simulink model "IOControls"  (R2019b)
settings: configuration reference "ConfigSet_IOControls_Reference" (kept outside this file)
model workspace (MAT data in the model file):
  SampleTime = 0.05
libraries: IOStateMachinesLib x274, SignalGeneratorsLib x1, simulink x1
(part 5 of 10)

== system IOControls/ForEachVehicle/IOControls/Non-CabControl/CircuitBreakersofEDB/BCGCB ==
  note: States:
      | Tripped
      | Set
  MCBControl : Inport  OutDataTypeStr=Bus: BD_IOControls_In_MCBControl
  Initialise : Inport  Port=2
  BCGCB-MCB : IOStateMachinesLib/MCB  InitSource=internal  InitState=InitState  OffStateValue=OffStateValue  OnStateValue=OnStateValue
      settings: SourceProductName=IO State Machines
  Bus Selector : BusSelector  OutputSignals=Value,Mode,InitVal,InternalRequest,Inhibit,TripRequest
  InputState : Outport  VectorParamsAs1DForOutWhenUnconnected=off
  MCBTripState : Outport  Port=2  VectorParamsAs1DForOutWhenUnconnected=off
  wires:
  BCGCB-MCB/2 -> MCBTripState/1
  Bus Selector/6 -> BCGCB-MCB/7  "<TripRequest>"
  MCBControl/1 -> Bus Selector/1
  Bus Selector/1 -> BCGCB-MCB/1  "<Value>"
  Bus Selector/2 -> BCGCB-MCB/2  "<Mode>"
  Bus Selector/3 -> BCGCB-MCB/3  "<InitVal>"
  Bus Selector/4 -> BCGCB-MCB/5  "<InternalRequest>"
  Bus Selector/5 -> BCGCB-MCB/6  "<Inhibit>"
  BCGCB-MCB/1 -> InputState/1
  Initialise/1 -> BCGCB-MCB/4

== system IOControls/ForEachVehicle/IOControls/Non-CabControl/CircuitBreakersofEDB/BECUCB1 ==
  note: States:
      | Tripped
      | Set
  MCBControl : Inport  OutDataTypeStr=Bus: BD_IOControls_In_MCBControl
  Initialise : Inport  Port=2
  BECUCB1-MCB : IOStateMachinesLib/MCB  InitSource=internal  InitState=InitState  OffStateValue=OffStateValue  OnStateValue=OnStateValue
      settings: SourceProductName=IO State Machines
  Bus Selector : BusSelector  OutputSignals=Value,Mode,InitVal,InternalRequest,Inhibit,TripRequest
  InputState : Outport  VectorParamsAs1DForOutWhenUnconnected=off
  MCBTripState : Outport  Port=2  VectorParamsAs1DForOutWhenUnconnected=off
  wires:
  BECUCB1-MCB/2 -> MCBTripState/1
  Bus Selector/6 -> BECUCB1-MCB/7  "<TripRequest>"
  MCBControl/1 -> Bus Selector/1
  Bus Selector/1 -> BECUCB1-MCB/1  "<Value>"
  Bus Selector/2 -> BECUCB1-MCB/2  "<Mode>"
  Bus Selector/3 -> BECUCB1-MCB/3  "<InitVal>"
  Bus Selector/4 -> BECUCB1-MCB/5  "<InternalRequest>"
  Bus Selector/5 -> BECUCB1-MCB/6  "<Inhibit>"
  BECUCB1-MCB/1 -> InputState/1
  Initialise/1 -> BECUCB1-MCB/4

== system IOControls/ForEachVehicle/IOControls/Non-CabControl/CircuitBreakersofEDB/BECUCB2 ==
  note: States:
      | Tripped
      | Set
  MCBControl : Inport  OutDataTypeStr=Bus: BD_IOControls_In_MCBControl
  Initialise : Inport  Port=2
  BECUCB2-MCB : IOStateMachinesLib/MCB  InitSource=internal  InitState=InitState  OffStateValue=OffStateValue  OnStateValue=OnStateValue
      settings: SourceProductName=IO State Machines
  Bus Selector : BusSelector  OutputSignals=Value,Mode,InitVal,InternalRequest,Inhibit,TripRequest
  InputState : Outport  VectorParamsAs1DForOutWhenUnconnected=off
  MCBTripState : Outport  Port=2  VectorParamsAs1DForOutWhenUnconnected=off
  wires:
  BECUCB2-MCB/2 -> MCBTripState/1
  Bus Selector/6 -> BECUCB2-MCB/7  "<TripRequest>"
  MCBControl/1 -> Bus Selector/1
  Bus Selector/1 -> BECUCB2-MCB/1  "<Value>"
  Bus Selector/2 -> BECUCB2-MCB/2  "<Mode>"
  Bus Selector/3 -> BECUCB2-MCB/3  "<InitVal>"
  Bus Selector/4 -> BECUCB2-MCB/5  "<InternalRequest>"
  Bus Selector/5 -> BECUCB2-MCB/6  "<Inhibit>"
  BECUCB2-MCB/1 -> InputState/1
  Initialise/1 -> BECUCB2-MCB/4

== system IOControls/ForEachVehicle/IOControls/Non-CabControl/CircuitBreakersofEDB/BECUCB3 ==
  note: States:
      | Tripped
      | Set
  MCBControl : Inport  OutDataTypeStr=Bus: BD_IOControls_In_MCBControl
  Initialise : Inport  Port=2
  BECUCB3-MCB : IOStateMachinesLib/MCB  InitSource=internal  InitState=InitState  OffStateValue=OffStateValue  OnStateValue=OnStateValue
      settings: SourceProductName=IO State Machines
  Bus Selector : BusSelector  OutputSignals=Value,Mode,InitVal,InternalRequest,Inhibit,TripRequest
  InputState : Outport  VectorParamsAs1DForOutWhenUnconnected=off
  MCBTripState : Outport  Port=2  VectorParamsAs1DForOutWhenUnconnected=off
  wires:
  BECUCB3-MCB/2 -> MCBTripState/1
  Bus Selector/6 -> BECUCB3-MCB/7  "<TripRequest>"
  MCBControl/1 -> Bus Selector/1
  Bus Selector/1 -> BECUCB3-MCB/1  "<Value>"
  Bus Selector/2 -> BECUCB3-MCB/2  "<Mode>"
  Bus Selector/3 -> BECUCB3-MCB/3  "<InitVal>"
  Bus Selector/4 -> BECUCB3-MCB/5  "<InternalRequest>"
  Bus Selector/5 -> BECUCB3-MCB/6  "<Inhibit>"
  BECUCB3-MCB/1 -> InputState/1
  Initialise/1 -> BECUCB3-MCB/4

== system IOControls/ForEachVehicle/IOControls/Non-CabControl/CircuitBreakersofEDB/BLCB ==
  note: States:
      | Tripped
      | Set
  MCBControl : Inport  OutDataTypeStr=Bus: BD_IOControls_In_MCBControl
  Initialise : Inport  Port=2
  BLCB-MCB : IOStateMachinesLib/MCB  InitSource=internal  InitState=InitState  OffStateValue=OffStateValue  OnStateValue=OnStateValue
      settings: SourceProductName=IO State Machines
  Bus Selector : BusSelector  OutputSignals=Value,Mode,InitVal,InternalRequest,Inhibit,TripRequest
  InputState : Outport  VectorParamsAs1DForOutWhenUnconnected=off
  MCBTripState : Outport  Port=2  VectorParamsAs1DForOutWhenUnconnected=off
  wires:
  BLCB-MCB/2 -> MCBTripState/1
  Bus Selector/6 -> BLCB-MCB/7  "<TripRequest>"
  MCBControl/1 -> Bus Selector/1
  Bus Selector/1 -> BLCB-MCB/1  "<Value>"
  Bus Selector/2 -> BLCB-MCB/2  "<Mode>"
  Bus Selector/3 -> BLCB-MCB/3  "<InitVal>"
  Bus Selector/4 -> BLCB-MCB/5  "<InternalRequest>"
  Bus Selector/5 -> BLCB-MCB/6  "<Inhibit>"
  BLCB-MCB/1 -> InputState/1
  Initialise/1 -> BLCB-MCB/4

== system IOControls/ForEachVehicle/IOControls/Non-CabControl/CircuitBreakersofEDB/C1CB ==
  note: States:
      | Tripped
      | Set
  MCBControl : Inport  OutDataTypeStr=Bus: BD_IOControls_In_MCBControl
  Initialise : Inport  Port=2
  Bus Selector : BusSelector  OutputSignals=Value,Mode,InitVal,InternalRequest,Inhibit,TripRequest
  C1CB-MCB : IOStateMachinesLib/MCB  InitSource=internal  InitState=InitState  OffStateValue=OffStateValue  OnStateValue=OnStateValue
      settings: SourceProductName=IO State Machines
  InputState : Outport  VectorParamsAs1DForOutWhenUnconnected=off
  MCBTripState : Outport  Port=2  VectorParamsAs1DForOutWhenUnconnected=off
  wires:
  C1CB-MCB/2 -> MCBTripState/1
  Bus Selector/6 -> C1CB-MCB/7  "<TripRequest>"
  MCBControl/1 -> Bus Selector/1
  Bus Selector/1 -> C1CB-MCB/1  "<Value>"
  Bus Selector/2 -> C1CB-MCB/2  "<Mode>"
  Bus Selector/3 -> C1CB-MCB/3  "<InitVal>"
  Bus Selector/4 -> C1CB-MCB/5  "<InternalRequest>"
  Bus Selector/5 -> C1CB-MCB/6  "<Inhibit>"
  C1CB-MCB/1 -> InputState/1
  Initialise/1 -> C1CB-MCB/4

== system IOControls/ForEachVehicle/IOControls/Non-CabControl/CircuitBreakersofEDB/CBFCB ==
  note: States:
      | Tripped
      | Set
  MCBControl : Inport  OutDataTypeStr=Bus: BD_IOControls_In_MCBControl
  Initialise : Inport  Port=2
  Bus Selector : BusSelector  OutputSignals=Value,Mode,InitVal,InternalRequest,Inhibit,TripRequest
  CBFCB-MCB : IOStateMachinesLib/MCB  InitSource=internal  InitState=InitState  OffStateValue=OffStateValue  OnStateValue=OnStateValue
      settings: SourceProductName=IO State Machines
  InputState : Outport  VectorParamsAs1DForOutWhenUnconnected=off
  MCBTripState : Outport  Port=2  VectorParamsAs1DForOutWhenUnconnected=off
  wires:
  CBFCB-MCB/2 -> MCBTripState/1
  Bus Selector/6 -> CBFCB-MCB/7  "<TripRequest>"
  MCBControl/1 -> Bus Selector/1
  Bus Selector/1 -> CBFCB-MCB/1  "<Value>"
  Bus Selector/2 -> CBFCB-MCB/2  "<Mode>"
  Bus Selector/3 -> CBFCB-MCB/3  "<InitVal>"
  Bus Selector/4 -> CBFCB-MCB/5  "<InternalRequest>"
  Bus Selector/5 -> CBFCB-MCB/6  "<Inhibit>"
  CBFCB-MCB/1 -> InputState/1
  Initialise/1 -> CBFCB-MCB/4

== system IOControls/ForEachVehicle/IOControls/Non-CabControl/CircuitBreakersofEDB/CBFCCB ==
  note: States:
      | Tripped
      | Set
  MCBControl : Inport  OutDataTypeStr=Bus: BD_IOControls_In_MCBControl
  Initialise : Inport  Port=2
  Bus Selector : BusSelector  OutputSignals=Value,Mode,InitVal,InternalRequest,Inhibit,TripRequest
  CBFCCB-MCB : IOStateMachinesLib/MCB  InitSource=internal  InitState=InitState  OffStateValue=OffStateValue  OnStateValue=OnStateValue
      settings: SourceProductName=IO State Machines
  InputState : Outport  VectorParamsAs1DForOutWhenUnconnected=off
  MCBTripState : Outport  Port=2  VectorParamsAs1DForOutWhenUnconnected=off
  wires:
  CBFCCB-MCB/2 -> MCBTripState/1
  Bus Selector/6 -> CBFCCB-MCB/7  "<TripRequest>"
  MCBControl/1 -> Bus Selector/1
  Bus Selector/1 -> CBFCCB-MCB/1  "<Value>"
  Bus Selector/2 -> CBFCCB-MCB/2  "<Mode>"
  Bus Selector/3 -> CBFCCB-MCB/3  "<InitVal>"
  Bus Selector/4 -> CBFCCB-MCB/5  "<InternalRequest>"
  Bus Selector/5 -> CBFCCB-MCB/6  "<Inhibit>"
  CBFCCB-MCB/1 -> InputState/1
  Initialise/1 -> CBFCCB-MCB/4

== system IOControls/ForEachVehicle/IOControls/Non-CabControl/CircuitBreakersofEDB/CBTCCB1 ==
  note: States:
      | Tripped
      | Set
  MCBControl : Inport  OutDataTypeStr=Bus: BD_IOControls_In_MCBControl
  Initialise : Inport  Port=2
  Bus Selector : BusSelector  OutputSignals=Value,Mode,InitVal,InternalRequest,Inhibit,TripRequest
  CBTCCB1-MCB : IOStateMachinesLib/MCB  InitSource=internal  InitState=InitState  OffStateValue=OffStateValue  OnStateValue=OnStateValue
      settings: SourceProductName=IO State Machines
  InputState : Outport  VectorParamsAs1DForOutWhenUnconnected=off
  MCBTripState : Outport  Port=2  VectorParamsAs1DForOutWhenUnconnected=off
  wires:
  CBTCCB1-MCB/2 -> MCBTripState/1
  Bus Selector/6 -> CBTCCB1-MCB/7  "<TripRequest>"
  MCBControl/1 -> Bus Selector/1
  Bus Selector/1 -> CBTCCB1-MCB/1  "<Value>"
  Bus Selector/2 -> CBTCCB1-MCB/2  "<Mode>"
  Bus Selector/3 -> CBTCCB1-MCB/3  "<InitVal>"
  Bus Selector/4 -> CBTCCB1-MCB/5  "<InternalRequest>"
  Bus Selector/5 -> CBTCCB1-MCB/6  "<Inhibit>"
  CBTCCB1-MCB/1 -> InputState/1
  Initialise/1 -> CBTCCB1-MCB/4

== system IOControls/ForEachVehicle/IOControls/Non-CabControl/CircuitBreakersofEDB/CCNVIO1CB ==
  note: States:
      | Tripped
      | Set
  MCBControl : Inport  OutDataTypeStr=Bus: BD_IOControls_In_MCBControl
  Initialise : Inport  Port=2
  Bus Selector : BusSelector  OutputSignals=Value,Mode,InitVal,InternalRequest,Inhibit,TripRequest
  CCNVIO1CB-MCB : IOStateMachinesLib/MCB  InitSource=internal  InitState=InitState  OffStateValue=OffStateValue  OnStateValue=OnStateValue
      settings: SourceProductName=IO State Machines
  InputState : Outport  VectorParamsAs1DForOutWhenUnconnected=off
  MCBTripState : Outport  Port=2  VectorParamsAs1DForOutWhenUnconnected=off
  wires:
  CCNVIO1CB-MCB/2 -> MCBTripState/1
  Bus Selector/6 -> CCNVIO1CB-MCB/7  "<TripRequest>"
  MCBControl/1 -> Bus Selector/1
  Bus Selector/1 -> CCNVIO1CB-MCB/1  "<Value>"
  Bus Selector/2 -> CCNVIO1CB-MCB/2  "<Mode>"
  Bus Selector/3 -> CCNVIO1CB-MCB/3  "<InitVal>"
  Bus Selector/4 -> CCNVIO1CB-MCB/5  "<InternalRequest>"
  Bus Selector/5 -> CCNVIO1CB-MCB/6  "<Inhibit>"
  CCNVIO1CB-MCB/1 -> InputState/1
  Initialise/1 -> CCNVIO1CB-MCB/4

== system IOControls/ForEachVehicle/IOControls/Non-CabControl/CircuitBreakersofEDB/CDUCB ==
  note: States:
      | Tripped
      | Set
  MCBControl : Inport  OutDataTypeStr=Bus: BD_IOControls_In_MCBControl
  Initialise : Inport  Port=2
  Bus Selector : BusSelector  OutputSignals=Value,Mode,InitVal,InternalRequest,Inhibit,TripRequest
  CDUCB-MCB : IOStateMachinesLib/MCB  InitSource=internal  InitState=InitState  OffStateValue=OffStateValue  OnStateValue=OnStateValue
      settings: SourceProductName=IO State Machines
  InputState : Outport  VectorParamsAs1DForOutWhenUnconnected=off
  MCBTripState : Outport  Port=2  VectorParamsAs1DForOutWhenUnconnected=off
  wires:
  CDUCB-MCB/2 -> MCBTripState/1
  Bus Selector/6 -> CDUCB-MCB/7  "<TripRequest>"
  MCBControl/1 -> Bus Selector/1
  Bus Selector/1 -> CDUCB-MCB/1  "<Value>"
  Bus Selector/2 -> CDUCB-MCB/2  "<Mode>"
  Bus Selector/3 -> CDUCB-MCB/3  "<InitVal>"
  Bus Selector/4 -> CDUCB-MCB/5  "<InternalRequest>"
  Bus Selector/5 -> CDUCB-MCB/6  "<Inhibit>"
  CDUCB-MCB/1 -> InputState/1
  Initialise/1 -> CDUCB-MCB/4

== system IOControls/ForEachVehicle/IOControls/Non-CabControl/CircuitBreakersofEDB/CECB ==
  note: States:
      | Tripped
      | Set
  MCBControl : Inport  OutDataTypeStr=Bus: BD_IOControls_In_MCBControl
  Initialise : Inport  Port=2
  Bus Selector : BusSelector  OutputSignals=Value,Mode,InitVal,InternalRequest,Inhibit,TripRequest
  CECB-MCB : IOStateMachinesLib/MCB  InitSource=internal  InitState=InitState  OffStateValue=OffStateValue  OnStateValue=OnStateValue
      settings: SourceProductName=IO State Machines
  InputState : Outport  VectorParamsAs1DForOutWhenUnconnected=off
  MCBTripState : Outport  Port=2  VectorParamsAs1DForOutWhenUnconnected=off
  wires:
  CECB-MCB/2 -> MCBTripState/1
  Bus Selector/6 -> CECB-MCB/7  "<TripRequest>"
  MCBControl/1 -> Bus Selector/1
  Bus Selector/1 -> CECB-MCB/1  "<Value>"
  Bus Selector/2 -> CECB-MCB/2  "<Mode>"
  Bus Selector/3 -> CECB-MCB/3  "<InitVal>"
  Bus Selector/4 -> CECB-MCB/5  "<InternalRequest>"
  Bus Selector/5 -> CECB-MCB/6  "<Inhibit>"
  CECB-MCB/1 -> InputState/1
  Initialise/1 -> CECB-MCB/4

== system IOControls/ForEachVehicle/IOControls/Non-CabControl/CircuitBreakersofEDB/CELCB ==
  note: States:
      | Tripped
      | Set
  MCBControl : Inport  OutDataTypeStr=Bus: BD_IOControls_In_MCBControl
  Initialise : Inport  Port=2
  Bus Selector : BusSelector  OutputSignals=Value,Mode,InitVal,InternalRequest,Inhibit,TripRequest
  CELCB-MCB : IOStateMachinesLib/MCB  InitSource=internal  InitState=InitState  OffStateValue=OffStateValue  OnStateValue=OnStateValue
      settings: SourceProductName=IO State Machines
  InputState : Outport  VectorParamsAs1DForOutWhenUnconnected=off
  MCBTripState : Outport  Port=2  VectorParamsAs1DForOutWhenUnconnected=off
  wires:
  CELCB-MCB/2 -> MCBTripState/1
  Bus Selector/6 -> CELCB-MCB/7  "<TripRequest>"
  MCBControl/1 -> Bus Selector/1
  Bus Selector/1 -> CELCB-MCB/1  "<Value>"
  Bus Selector/2 -> CELCB-MCB/2  "<Mode>"
  Bus Selector/3 -> CELCB-MCB/3  "<InitVal>"
  Bus Selector/4 -> CELCB-MCB/5  "<InternalRequest>"
  Bus Selector/5 -> CELCB-MCB/6  "<Inhibit>"
  CELCB-MCB/1 -> InputState/1
  Initialise/1 -> CELCB-MCB/4

== system IOControls/ForEachVehicle/IOControls/Non-CabControl/CircuitBreakersofEDB/CICB ==
  note: States:
      | Tripped
      | Set
  MCBControl : Inport  OutDataTypeStr=Bus: BD_IOControls_In_MCBControl
  Initialise : Inport  Port=2
  Bus Selector : BusSelector  OutputSignals=Value,Mode,InitVal,InternalRequest,Inhibit,TripRequest
  CICB-MCB : IOStateMachinesLib/MCB  InitSource=internal  InitState=InitState  OffStateValue=OffStateValue  OnStateValue=OnStateValue
      settings: SourceProductName=IO State Machines
  InputState : Outport  VectorParamsAs1DForOutWhenUnconnected=off
  MCBTripState : Outport  Port=2  VectorParamsAs1DForOutWhenUnconnected=off
  wires:
  CICB-MCB/2 -> MCBTripState/1
  Bus Selector/6 -> CICB-MCB/7  "<TripRequest>"
  MCBControl/1 -> Bus Selector/1
  Bus Selector/1 -> CICB-MCB/1  "<Value>"
  Bus Selector/2 -> CICB-MCB/2  "<Mode>"
  Bus Selector/3 -> CICB-MCB/3  "<InitVal>"
  Bus Selector/4 -> CICB-MCB/5  "<InternalRequest>"
  Bus Selector/5 -> CICB-MCB/6  "<Inhibit>"
  CICB-MCB/1 -> InputState/1
  Initialise/1 -> CICB-MCB/4

== system IOControls/ForEachVehicle/IOControls/Non-CabControl/CircuitBreakersofEDB/CILCB ==
  note: States:
      | Tripped
      | Set
  MCBControl : Inport  OutDataTypeStr=Bus: BD_IOControls_In_MCBControl
  Initialise : Inport  Port=2
  Bus Selector : BusSelector  OutputSignals=Value,Mode,InitVal,InternalRequest,Inhibit,TripRequest
  CILCB-MCB : IOStateMachinesLib/MCB  InitSource=internal  InitState=InitState  OffStateValue=OffStateValue  OnStateValue=OnStateValue
      settings: SourceProductName=IO State Machines
  InputState : Outport  VectorParamsAs1DForOutWhenUnconnected=off
  MCBTripState : Outport  Port=2  VectorParamsAs1DForOutWhenUnconnected=off
  wires:
  CILCB-MCB/2 -> MCBTripState/1
  Bus Selector/6 -> CILCB-MCB/7  "<TripRequest>"
  MCBControl/1 -> Bus Selector/1
  Bus Selector/1 -> CILCB-MCB/1  "<Value>"
  Bus Selector/2 -> CILCB-MCB/2  "<Mode>"
  Bus Selector/3 -> CILCB-MCB/3  "<InitVal>"
  Bus Selector/4 -> CILCB-MCB/5  "<InternalRequest>"
  Bus Selector/5 -> CILCB-MCB/6  "<Inhibit>"
  CILCB-MCB/1 -> InputState/1
  Initialise/1 -> CILCB-MCB/4

== system IOControls/ForEachVehicle/IOControls/Non-CabControl/CircuitBreakersofEDB/CMCB ==
  note: States:
      | Tripped
      | Set
  MCBControl : Inport  OutDataTypeStr=Bus: BD_IOControls_In_MCBControl
  Initialise : Inport  Port=2
  Bus Selector : BusSelector  OutputSignals=Value,Mode,InitVal,InternalRequest,Inhibit,TripRequest
  CMCB-MCB : IOStateMachinesLib/MCB  InitSource=internal  InitState=InitState  OffStateValue=OffStateValue  OnStateValue=OnStateValue
      settings: SourceProductName=IO State Machines
  InputState : Outport  VectorParamsAs1DForOutWhenUnconnected=off
  MCBTripState : Outport  Port=2  VectorParamsAs1DForOutWhenUnconnected=off
  wires:
  CMCB-MCB/2 -> MCBTripState/1
  Bus Selector/6 -> CMCB-MCB/7  "<TripRequest>"
  MCBControl/1 -> Bus Selector/1
  Bus Selector/1 -> CMCB-MCB/1  "<Value>"
  Bus Selector/2 -> CMCB-MCB/2  "<Mode>"
  Bus Selector/3 -> CMCB-MCB/3  "<InitVal>"
  Bus Selector/4 -> CMCB-MCB/5  "<InternalRequest>"
  Bus Selector/5 -> CMCB-MCB/6  "<Inhibit>"
  CMCB-MCB/1 -> InputState/1
  Initialise/1 -> CMCB-MCB/4

== system IOControls/ForEachVehicle/IOControls/Non-CabControl/CircuitBreakersofEDB/CMCCB ==
  note: States:
      | Tripped
      | Set
  MCBControl : Inport  OutDataTypeStr=Bus: BD_IOControls_In_MCBControl
  Initialise : Inport  Port=2
  Bus Selector : BusSelector  OutputSignals=Value,Mode,InitVal,InternalRequest,Inhibit,TripRequest
  CMCCB-MCB : IOStateMachinesLib/MCB  InitSource=internal  InitState=InitState  OffStateValue=OffStateValue  OnStateValue=OnStateValue
      settings: SourceProductName=IO State Machines
  InputState : Outport  VectorParamsAs1DForOutWhenUnconnected=off
  MCBTripState : Outport  Port=2  VectorParamsAs1DForOutWhenUnconnected=off
  wires:
  CMCCB-MCB/2 -> MCBTripState/1
  Bus Selector/6 -> CMCCB-MCB/7  "<TripRequest>"
  MCBControl/1 -> Bus Selector/1
  Bus Selector/1 -> CMCCB-MCB/1  "<Value>"
  Bus Selector/2 -> CMCCB-MCB/2  "<Mode>"
  Bus Selector/3 -> CMCCB-MCB/3  "<InitVal>"
  Bus Selector/4 -> CMCCB-MCB/5  "<InternalRequest>"
  Bus Selector/5 -> CMCCB-MCB/6  "<Inhibit>"
  CMCCB-MCB/1 -> InputState/1
  Initialise/1 -> CMCCB-MCB/4

== system IOControls/ForEachVehicle/IOControls/Non-CabControl/CircuitBreakersofEDB/CRSBCB ==
  note: States:
      | Tripped
      | Set
  MCBControl : Inport  OutDataTypeStr=Bus: BD_IOControls_In_MCBControl
  Initialise : Inport  Port=2
  Bus Selector : BusSelector  OutputSignals=Value,Mode,InitVal,InternalRequest,Inhibit,TripRequest
  CRSBCB-MCB : IOStateMachinesLib/MCB  InitSource=internal  InitState=InitState  OffStateValue=OffStateValue  OnStateValue=OnStateValue
      settings: SourceProductName=IO State Machines
  InputState : Outport  VectorParamsAs1DForOutWhenUnconnected=off
  MCBTripState : Outport  Port=2  VectorParamsAs1DForOutWhenUnconnected=off
  wires:
  CRSBCB-MCB/2 -> MCBTripState/1
  Bus Selector/6 -> CRSBCB-MCB/7  "<TripRequest>"
  MCBControl/1 -> Bus Selector/1
  Bus Selector/1 -> CRSBCB-MCB/1  "<Value>"
  Bus Selector/2 -> CRSBCB-MCB/2  "<Mode>"
  Bus Selector/3 -> CRSBCB-MCB/3  "<InitVal>"
  Bus Selector/4 -> CRSBCB-MCB/5  "<InternalRequest>"
  Bus Selector/5 -> CRSBCB-MCB/6  "<Inhibit>"
  CRSBCB-MCB/1 -> InputState/1
  Initialise/1 -> CRSBCB-MCB/4

== system IOControls/ForEachVehicle/IOControls/Non-CabControl/CircuitBreakersofEDB/CSACB ==
  note: States:
      | Tripped
      | Set
  MCBControl : Inport  OutDataTypeStr=Bus: BD_IOControls_In_MCBControl
  Initialise : Inport  Port=2
  Bus Selector : BusSelector  OutputSignals=Value,Mode,InitVal,InternalRequest,Inhibit,TripRequest
  CSACB-MCB : IOStateMachinesLib/MCB  InitSource=internal  InitState=InitState  OffStateValue=OffStateValue  OnStateValue=OnStateValue
      settings: SourceProductName=IO State Machines
  InputState : Outport  VectorParamsAs1DForOutWhenUnconnected=off
  MCBTripState : Outport  Port=2  VectorParamsAs1DForOutWhenUnconnected=off
  wires:
  CSACB-MCB/2 -> MCBTripState/1
  Bus Selector/6 -> CSACB-MCB/7  "<TripRequest>"
  MCBControl/1 -> Bus Selector/1
  Bus Selector/1 -> CSACB-MCB/1  "<Value>"
  Bus Selector/2 -> CSACB-MCB/2  "<Mode>"
  Bus Selector/3 -> CSACB-MCB/3  "<InitVal>"
  Bus Selector/4 -> CSACB-MCB/5  "<InternalRequest>"
  Bus Selector/5 -> CSACB-MCB/6  "<Inhibit>"
  CSACB-MCB/1 -> InputState/1
  Initialise/1 -> CSACB-MCB/4

== system IOControls/ForEachVehicle/IOControls/Non-CabControl/CircuitBreakersofEDB/CSBCB ==
  note: States:
      | Tripped
      | Set
  MCBControl : Inport  OutDataTypeStr=Bus: BD_IOControls_In_MCBControl
  Initialise : Inport  Port=2
  Bus Selector : BusSelector  OutputSignals=Value,Mode,InitVal,InternalRequest,Inhibit,TripRequest
  CSBCB-MCB : IOStateMachinesLib/MCB  InitSource=internal  InitState=InitState  OffStateValue=OffStateValue  OnStateValue=OnStateValue
      settings: SourceProductName=IO State Machines
  InputState : Outport  VectorParamsAs1DForOutWhenUnconnected=off
  MCBTripState : Outport  Port=2  VectorParamsAs1DForOutWhenUnconnected=off
  wires:
  CSBCB-MCB/2 -> MCBTripState/1
  Bus Selector/6 -> CSBCB-MCB/7  "<TripRequest>"
  MCBControl/1 -> Bus Selector/1
  Bus Selector/1 -> CSBCB-MCB/1  "<Value>"
  Bus Selector/2 -> CSBCB-MCB/2  "<Mode>"
  Bus Selector/3 -> CSBCB-MCB/3  "<InitVal>"
  Bus Selector/4 -> CSBCB-MCB/5  "<InternalRequest>"
  Bus Selector/5 -> CSBCB-MCB/6  "<Inhibit>"
  CSBCB-MCB/1 -> InputState/1
  Initialise/1 -> CSBCB-MCB/4

== system IOControls/ForEachVehicle/IOControls/Non-CabControl/CircuitBreakersofEDB/CSCCB ==
  note: States:
      | Tripped
      | Set
  MCBControl : Inport  OutDataTypeStr=Bus: BD_IOControls_In_MCBControl
  Initialise : Inport  Port=2
  Bus Selector : BusSelector  OutputSignals=Value,Mode,InitVal,InternalRequest,Inhibit,TripRequest
  CSCCB-MCB : IOStateMachinesLib/MCB  InitSource=internal  InitState=InitState  OffStateValue=OffStateValue  OnStateValue=OnStateValue
      settings: SourceProductName=IO State Machines
  InputState : Outport  VectorParamsAs1DForOutWhenUnconnected=off
  MCBTripState : Outport  Port=2  VectorParamsAs1DForOutWhenUnconnected=off
  wires:
  CSCCB-MCB/2 -> MCBTripState/1
  Bus Selector/6 -> CSCCB-MCB/7  "<TripRequest>"
  MCBControl/1 -> Bus Selector/1
  Bus Selector/1 -> CSCCB-MCB/1  "<Value>"
  Bus Selector/2 -> CSCCB-MCB/2  "<Mode>"
  Bus Selector/3 -> CSCCB-MCB/3  "<InitVal>"
  Bus Selector/4 -> CSCCB-MCB/5  "<InternalRequest>"
  Bus Selector/5 -> CSCCB-MCB/6  "<Inhibit>"
  CSCCB-MCB/1 -> InputState/1
  Initialise/1 -> CSCCB-MCB/4

== system IOControls/ForEachVehicle/IOControls/Non-CabControl/CircuitBreakersofEDB/DIOCB1 ==
  note: States:
      | Tripped
      | Set
  MCBControl : Inport  OutDataTypeStr=Bus: BD_IOControls_In_MCBControl
  Initialise : Inport  Port=2
  Bus Selector : BusSelector  OutputSignals=Value,Mode,InitVal,InternalRequest,Inhibit,TripRequest
  DIOCB1-MCB : IOStateMachinesLib/MCB  InitSource=internal  InitState=InitState  OffStateValue=OffStateValue  OnStateValue=OnStateValue
      settings: SourceProductName=IO State Machines
  InputState : Outport  VectorParamsAs1DForOutWhenUnconnected=off
  MCBTripState : Outport  Port=2  VectorParamsAs1DForOutWhenUnconnected=off
  wires:
  DIOCB1-MCB/2 -> MCBTripState/1
  Bus Selector/6 -> DIOCB1-MCB/7  "<TripRequest>"
  MCBControl/1 -> Bus Selector/1
  Bus Selector/1 -> DIOCB1-MCB/1  "<Value>"
  Bus Selector/2 -> DIOCB1-MCB/2  "<Mode>"
  Bus Selector/3 -> DIOCB1-MCB/3  "<InitVal>"
  Bus Selector/4 -> DIOCB1-MCB/5  "<InternalRequest>"
  Bus Selector/5 -> DIOCB1-MCB/6  "<Inhibit>"
  DIOCB1-MCB/1 -> InputState/1
  Initialise/1 -> DIOCB1-MCB/4

== system IOControls/ForEachVehicle/IOControls/Non-CabControl/CircuitBreakersofEDB/DIOCB2 ==
  note: States:
      | Tripped
      | Set
  MCBControl : Inport  OutDataTypeStr=Bus: BD_IOControls_In_MCBControl
  Initialise : Inport  Port=2
  Bus Selector : BusSelector  OutputSignals=Value,Mode,InitVal,InternalRequest,Inhibit,TripRequest
  DIOCB2-MCB : IOStateMachinesLib/MCB  InitSource=internal  InitState=InitState  OffStateValue=OffStateValue  OnStateValue=OnStateValue
      settings: SourceProductName=IO State Machines
  InputState : Outport  VectorParamsAs1DForOutWhenUnconnected=off
  MCBTripState : Outport  Port=2  VectorParamsAs1DForOutWhenUnconnected=off
  wires:
  DIOCB2-MCB/2 -> MCBTripState/1
  Bus Selector/6 -> DIOCB2-MCB/7  "<TripRequest>"
  MCBControl/1 -> Bus Selector/1
  Bus Selector/1 -> DIOCB2-MCB/1  "<Value>"
  Bus Selector/2 -> DIOCB2-MCB/2  "<Mode>"
  Bus Selector/3 -> DIOCB2-MCB/3  "<InitVal>"
  Bus Selector/4 -> DIOCB2-MCB/5  "<InternalRequest>"
  Bus Selector/5 -> DIOCB2-MCB/6  "<Inhibit>"
  DIOCB2-MCB/1 -> InputState/1
  Initialise/1 -> DIOCB2-MCB/4

== system IOControls/ForEachVehicle/IOControls/Non-CabControl/CircuitBreakersofEDB/DLCB ==
  note: States:
      | Tripped
      | Set
  MCBControl : Inport  OutDataTypeStr=Bus: BD_IOControls_In_MCBControl
  Initialise : Inport  Port=2
  Bus Selector : BusSelector  OutputSignals=Value,Mode,InitVal,InternalRequest,Inhibit,TripRequest
  DLCB-MCB : IOStateMachinesLib/MCB  InitSource=internal  InitState=InitState  OffStateValue=OffStateValue  OnStateValue=OnStateValue
      settings: SourceProductName=IO State Machines
  InputState : Outport  VectorParamsAs1DForOutWhenUnconnected=off
  MCBTripState : Outport  Port=2  VectorParamsAs1DForOutWhenUnconnected=off
  wires:
  DLCB-MCB/2 -> MCBTripState/1
  Bus Selector/6 -> DLCB-MCB/7  "<TripRequest>"
  MCBControl/1 -> Bus Selector/1
  Bus Selector/1 -> DLCB-MCB/1  "<Value>"
  Bus Selector/2 -> DLCB-MCB/2  "<Mode>"
  Bus Selector/3 -> DLCB-MCB/3  "<InitVal>"
  Bus Selector/4 -> DLCB-MCB/5  "<InternalRequest>"
  Bus Selector/5 -> DLCB-MCB/6  "<Inhibit>"
  DLCB-MCB/1 -> InputState/1
  Initialise/1 -> DLCB-MCB/4

== system IOControls/ForEachVehicle/IOControls/Non-CabControl/CircuitBreakersofEDB/DMICB ==
  note: States:
      | Tripped
      | Set
  MCBControl : Inport  OutDataTypeStr=Bus: BD_IOControls_In_MCBControl
  Initialise : Inport  Port=2
  Bus Selector : BusSelector  OutputSignals=Value,Mode,InitVal,InternalRequest,Inhibit,TripRequest
  DMICB-MCB : IOStateMachinesLib/MCB  InitSource=internal  InitState=InitState  OffStateValue=OffStateValue  OnStateValue=OnStateValue
      settings: SourceProductName=IO State Machines
  InputState : Outport  VectorParamsAs1DForOutWhenUnconnected=off
  MCBTripState : Outport  Port=2  VectorParamsAs1DForOutWhenUnconnected=off
  wires:
  DMICB-MCB/2 -> MCBTripState/1
  Bus Selector/6 -> DMICB-MCB/7  "<TripRequest>"
  MCBControl/1 -> Bus Selector/1
  Bus Selector/1 -> DMICB-MCB/1  "<Value>"
  Bus Selector/2 -> DMICB-MCB/2  "<Mode>"
  Bus Selector/3 -> DMICB-MCB/3  "<InitVal>"
  Bus Selector/4 -> DMICB-MCB/5  "<InternalRequest>"
  Bus Selector/5 -> DMICB-MCB/6  "<Inhibit>"
  DMICB-MCB/1 -> InputState/1
  Initialise/1 -> DMICB-MCB/4

== system IOControls/ForEachVehicle/IOControls/Non-CabControl/CircuitBreakersofEDB/DPLCB ==
  note: States:
      | Tripped
      | Set
  MCBControl : Inport  OutDataTypeStr=Bus: BD_IOControls_In_MCBControl
  Initialise : Inport  Port=2
  Bus Selector : BusSelector  OutputSignals=Value,Mode,InitVal,InternalRequest,Inhibit,TripRequest
  DPLCB-MCB : IOStateMachinesLib/MCB  InitSource=internal  InitState=InitState  OffStateValue=OffStateValue  OnStateValue=OnStateValue
      settings: SourceProductName=IO State Machines
  InputState : Outport  VectorParamsAs1DForOutWhenUnconnected=off
  MCBTripState : Outport  Port=2  VectorParamsAs1DForOutWhenUnconnected=off
  wires:
  DPLCB-MCB/2 -> MCBTripState/1
  Bus Selector/6 -> DPLCB-MCB/7  "<TripRequest>"
  MCBControl/1 -> Bus Selector/1
  Bus Selector/1 -> DPLCB-MCB/1  "<Value>"
  Bus Selector/2 -> DPLCB-MCB/2  "<Mode>"
  Bus Selector/3 -> DPLCB-MCB/3  "<InitVal>"
  Bus Selector/4 -> DPLCB-MCB/5  "<InternalRequest>"
  Bus Selector/5 -> DPLCB-MCB/6  "<Inhibit>"
  DPLCB-MCB/1 -> InputState/1
  Initialise/1 -> DPLCB-MCB/4

== system IOControls/ForEachVehicle/IOControls/Non-CabControl/CircuitBreakersofEDB/DRCB ==
  note: States:
      | Tripped
      | Set
  MCBControl : Inport  OutDataTypeStr=Bus: BD_IOControls_In_MCBControl
  Initialise : Inport  Port=2
  Bus Selector : BusSelector  OutputSignals=Value,Mode,InitVal,InternalRequest,Inhibit,TripRequest
  DRCB-MCB : IOStateMachinesLib/MCB  InitSource=internal  InitState=InitState  OffStateValue=OffStateValue  OnStateValue=OnStateValue
      settings: SourceProductName=IO State Machines
  InputState : Outport  VectorParamsAs1DForOutWhenUnconnected=off
  MCBTripState : Outport  Port=2  VectorParamsAs1DForOutWhenUnconnected=off
  wires:
  DRCB-MCB/2 -> MCBTripState/1
  Bus Selector/6 -> DRCB-MCB/7  "<TripRequest>"
  MCBControl/1 -> Bus Selector/1
  Bus Selector/1 -> DRCB-MCB/1  "<Value>"
  Bus Selector/2 -> DRCB-MCB/2  "<Mode>"
  Bus Selector/3 -> DRCB-MCB/3  "<InitVal>"
  Bus Selector/4 -> DRCB-MCB/5  "<InternalRequest>"
  Bus Selector/5 -> DRCB-MCB/6  "<Inhibit>"
  DRCB-MCB/1 -> InputState/1
  Initialise/1 -> DRCB-MCB/4

== system IOControls/ForEachVehicle/IOControls/Non-CabControl/CircuitBreakersofEDB/DSCB ==
  note: States:
      | Tripped
      | Set
  MCBControl : Inport  OutDataTypeStr=Bus: BD_IOControls_In_MCBControl
  Initialise : Inport  Port=2
  Bus Selector : BusSelector  OutputSignals=Value,Mode,InitVal,InternalRequest,Inhibit,TripRequest
  DSCB-MCB : IOStateMachinesLib/MCB  InitSource=internal  InitState=InitState  OffStateValue=OffStateValue  OnStateValue=OnStateValue
      settings: SourceProductName=IO State Machines
  InputState : Outport  VectorParamsAs1DForOutWhenUnconnected=off
  MCBTripState : Outport  Port=2  VectorParamsAs1DForOutWhenUnconnected=off
  wires:
  DSCB-MCB/2 -> MCBTripState/1
  Bus Selector/6 -> DSCB-MCB/7  "<TripRequest>"
  MCBControl/1 -> Bus Selector/1
  Bus Selector/1 -> DSCB-MCB/1  "<Value>"
  Bus Selector/2 -> DSCB-MCB/2  "<Mode>"
  Bus Selector/3 -> DSCB-MCB/3  "<InitVal>"
  Bus Selector/4 -> DSCB-MCB/5  "<InternalRequest>"
  Bus Selector/5 -> DSCB-MCB/6  "<Inhibit>"
  DSCB-MCB/1 -> InputState/1
  Initialise/1 -> DSCB-MCB/4

== system IOControls/ForEachVehicle/IOControls/Non-CabControl/CircuitBreakersofEDB/EBLR1CB ==
  note: States:
      | Tripped
      | Set
  MCBControl : Inport  OutDataTypeStr=Bus: BD_IOControls_In_MCBControl
  Initialise : Inport  Port=2
  Bus Selector : BusSelector  OutputSignals=Value,Mode,InitVal,InternalRequest,Inhibit,TripRequest
  EBLR1CB-MCB : IOStateMachinesLib/MCB  InitSource=internal  InitState=InitState  OffStateValue=OffStateValue  OnStateValue=OnStateValue
      settings: SourceProductName=IO State Machines
  InputState : Outport  VectorParamsAs1DForOutWhenUnconnected=off
  MCBTripState : Outport  Port=2  VectorParamsAs1DForOutWhenUnconnected=off
  wires:
  EBLR1CB-MCB/2 -> MCBTripState/1
  Bus Selector/6 -> EBLR1CB-MCB/7  "<TripRequest>"
  MCBControl/1 -> Bus Selector/1
  Bus Selector/1 -> EBLR1CB-MCB/1  "<Value>"
  Bus Selector/2 -> EBLR1CB-MCB/2  "<Mode>"
  Bus Selector/3 -> EBLR1CB-MCB/3  "<InitVal>"
  Bus Selector/4 -> EBLR1CB-MCB/5  "<InternalRequest>"
  Bus Selector/5 -> EBLR1CB-MCB/6  "<Inhibit>"
  EBLR1CB-MCB/1 -> InputState/1
  Initialise/1 -> EBLR1CB-MCB/4

== system IOControls/ForEachVehicle/IOControls/Non-CabControl/CircuitBreakersofEDB/EBLR2CB ==
  note: States:
      | Tripped
      | Set
  MCBControl : Inport  OutDataTypeStr=Bus: BD_IOControls_In_MCBControl
  Initialise : Inport  Port=2
  Bus Selector : BusSelector  OutputSignals=Value,Mode,InitVal,InternalRequest,Inhibit,TripRequest
  EBLR2CB-MCB : IOStateMachinesLib/MCB  InitSource=internal  InitState=InitState  OffStateValue=OffStateValue  OnStateValue=OnStateValue
      settings: SourceProductName=IO State Machines
  InputState : Outport  VectorParamsAs1DForOutWhenUnconnected=off
  MCBTripState : Outport  Port=2  VectorParamsAs1DForOutWhenUnconnected=off
  wires:
  EBLR2CB-MCB/2 -> MCBTripState/1
  Bus Selector/6 -> EBLR2CB-MCB/7  "<TripRequest>"
  MCBControl/1 -> Bus Selector/1
  Bus Selector/1 -> EBLR2CB-MCB/1  "<Value>"
  Bus Selector/2 -> EBLR2CB-MCB/2  "<Mode>"
  Bus Selector/3 -> EBLR2CB-MCB/3  "<InitVal>"
  Bus Selector/4 -> EBLR2CB-MCB/5  "<InternalRequest>"
  Bus Selector/5 -> EBLR2CB-MCB/6  "<Inhibit>"
  EBLR2CB-MCB/1 -> InputState/1
  Initialise/1 -> EBLR2CB-MCB/4

== system IOControls/ForEachVehicle/IOControls/Non-CabControl/CircuitBreakersofEDB/EBMVCB ==
  note: States:
      | Tripped
      | Set
  MCBControl : Inport  OutDataTypeStr=Bus: BD_IOControls_In_MCBControl
  Initialise : Inport  Port=2
  Bus Selector : BusSelector  OutputSignals=Value,Mode,InitVal,InternalRequest,Inhibit,TripRequest
  EBMVCB-MCB : IOStateMachinesLib/MCB  InitSource=internal  InitState=InitState  OffStateValue=OffStateValue  OnStateValue=OnStateValue
      settings: SourceProductName=IO State Machines
  InputState : Outport  VectorParamsAs1DForOutWhenUnconnected=off
  MCBTripState : Outport  Port=2  VectorParamsAs1DForOutWhenUnconnected=off
  wires:
  EBMVCB-MCB/2 -> MCBTripState/1
  Bus Selector/6 -> EBMVCB-MCB/7  "<TripRequest>"
  MCBControl/1 -> Bus Selector/1
  Bus Selector/1 -> EBMVCB-MCB/1  "<Value>"
  Bus Selector/2 -> EBMVCB-MCB/2  "<Mode>"
  Bus Selector/3 -> EBMVCB-MCB/3  "<InitVal>"
  Bus Selector/4 -> EBMVCB-MCB/5  "<InternalRequest>"
  Bus Selector/5 -> EBMVCB-MCB/6  "<Inhibit>"
  EBMVCB-MCB/1 -> InputState/1
  Initialise/1 -> EBMVCB-MCB/4

== system IOControls/ForEachVehicle/IOControls/Non-CabControl/CircuitBreakersofEDB/EDCB ==
  note: States:
      | Tripped
      | Set
  MCBControl : Inport  OutDataTypeStr=Bus: BD_IOControls_In_MCBControl
  Initialise : Inport  Port=2
  Bus Selector : BusSelector  OutputSignals=Value,Mode,InitVal,InternalRequest,Inhibit,TripRequest
  EDCB-MCB : IOStateMachinesLib/MCB  InitSource=internal  InitState=InitState  OffStateValue=OffStateValue  OnStateValue=OnStateValue
      settings: SourceProductName=IO State Machines
  InputState : Outport  VectorParamsAs1DForOutWhenUnconnected=off
  MCBTripState : Outport  Port=2  VectorParamsAs1DForOutWhenUnconnected=off
  wires:
  EDCB-MCB/2 -> MCBTripState/1
  Bus Selector/6 -> EDCB-MCB/7  "<TripRequest>"
  MCBControl/1 -> Bus Selector/1
  Bus Selector/1 -> EDCB-MCB/1  "<Value>"
  Bus Selector/2 -> EDCB-MCB/2  "<Mode>"
  Bus Selector/3 -> EDCB-MCB/3  "<InitVal>"
  Bus Selector/4 -> EDCB-MCB/5  "<InternalRequest>"
  Bus Selector/5 -> EDCB-MCB/6  "<Inhibit>"
  EDCB-MCB/1 -> InputState/1
  Initialise/1 -> EDCB-MCB/4

== system IOControls/ForEachVehicle/IOControls/Non-CabControl/CircuitBreakersofEDB/ELCB1 ==
  note: States:
      | Tripped
      | Set
  MCBControl : Inport  OutDataTypeStr=Bus: BD_IOControls_In_MCBControl
  Initialise : Inport  Port=2
  Bus Selector : BusSelector  OutputSignals=Value,Mode,InitVal,InternalRequest,Inhibit,TripRequest
  ELCB1-MCB : IOStateMachinesLib/MCB  InitSource=internal  InitState=InitState  OffStateValue=OffStateValue  OnStateValue=OnStateValue
      settings: SourceProductName=IO State Machines
  InputState : Outport  VectorParamsAs1DForOutWhenUnconnected=off
  MCBTripState : Outport  Port=2  VectorParamsAs1DForOutWhenUnconnected=off
  wires:
  ELCB1-MCB/2 -> MCBTripState/1
  Bus Selector/6 -> ELCB1-MCB/7  "<TripRequest>"
  MCBControl/1 -> Bus Selector/1
  Bus Selector/1 -> ELCB1-MCB/1  "<Value>"
  Bus Selector/2 -> ELCB1-MCB/2  "<Mode>"
  Bus Selector/3 -> ELCB1-MCB/3  "<InitVal>"
  Bus Selector/4 -> ELCB1-MCB/5  "<InternalRequest>"
  Bus Selector/5 -> ELCB1-MCB/6  "<Inhibit>"
  ELCB1-MCB/1 -> InputState/1
  Initialise/1 -> ELCB1-MCB/4

== system IOControls/ForEachVehicle/IOControls/Non-CabControl/CircuitBreakersofEDB/ELCB2 ==
  note: States:
      | Tripped
      | Set
  MCBControl : Inport  OutDataTypeStr=Bus: BD_IOControls_In_MCBControl
  Initialise : Inport  Port=2
  Bus Selector : BusSelector  OutputSignals=Value,Mode,InitVal,InternalRequest,Inhibit,TripRequest
  ELCB2-MCB : IOStateMachinesLib/MCB  InitSource=internal  InitState=InitState  OffStateValue=OffStateValue  OnStateValue=OnStateValue
      settings: SourceProductName=IO State Machines
  InputState : Outport  VectorParamsAs1DForOutWhenUnconnected=off
  MCBTripState : Outport  Port=2  VectorParamsAs1DForOutWhenUnconnected=off
  wires:
  ELCB2-MCB/2 -> MCBTripState/1
  Bus Selector/6 -> ELCB2-MCB/7  "<TripRequest>"
  MCBControl/1 -> Bus Selector/1
  Bus Selector/1 -> ELCB2-MCB/1  "<Value>"
  Bus Selector/2 -> ELCB2-MCB/2  "<Mode>"
  Bus Selector/3 -> ELCB2-MCB/3  "<InitVal>"
  Bus Selector/4 -> ELCB2-MCB/5  "<InternalRequest>"
  Bus Selector/5 -> ELCB2-MCB/6  "<Inhibit>"
  ELCB2-MCB/1 -> InputState/1
  Initialise/1 -> ELCB2-MCB/4

== system IOControls/ForEachVehicle/IOControls/Non-CabControl/CircuitBreakersofEDB/ERCB ==
  note: States:
      | Tripped
      | Set
  MCBControl : Inport  OutDataTypeStr=Bus: BD_IOControls_In_MCBControl
  Initialise : Inport  Port=2
  Bus Selector : BusSelector  OutputSignals=Value,Mode,InitVal,InternalRequest,Inhibit,TripRequest
  ERCB-MCB : IOStateMachinesLib/MCB  InitSource=internal  InitState=InitState  OffStateValue=OffStateValue  OnStateValue=OnStateValue
      settings: SourceProductName=IO State Machines
  InputState : Outport  VectorParamsAs1DForOutWhenUnconnected=off
  MCBTripState : Outport  Port=2  VectorParamsAs1DForOutWhenUnconnected=off
  wires:
  ERCB-MCB/2 -> MCBTripState/1
  Bus Selector/6 -> ERCB-MCB/7  "<TripRequest>"
  MCBControl/1 -> Bus Selector/1
  Bus Selector/1 -> ERCB-MCB/1  "<Value>"
  Bus Selector/2 -> ERCB-MCB/2  "<Mode>"
  Bus Selector/3 -> ERCB-MCB/3  "<InitVal>"
  Bus Selector/4 -> ERCB-MCB/5  "<InternalRequest>"
  Bus Selector/5 -> ERCB-MCB/6  "<Inhibit>"
  ERCB-MCB/1 -> InputState/1
  Initialise/1 -> ERCB-MCB/4

== system IOControls/ForEachVehicle/IOControls/Non-CabControl/CircuitBreakersofEDB/ERVRCB1 ==
  note: States:
      | Tripped
      | Set
  MCBControl : Inport  OutDataTypeStr=Bus: BD_IOControls_In_MCBControl
  Initialise : Inport  Port=2
  Bus Selector : BusSelector  OutputSignals=Value,Mode,InitVal,InternalRequest,Inhibit,TripRequest
  ERVRCB1-MCB : IOStateMachinesLib/MCB  InitSource=internal  InitState=InitState  OffStateValue=OffStateValue  OnStateValue=OnStateValue
      settings: SourceProductName=IO State Machines
  InputState : Outport  VectorParamsAs1DForOutWhenUnconnected=off
  MCBTripState : Outport  Port=2  VectorParamsAs1DForOutWhenUnconnected=off
  wires:
  ERVRCB1-MCB/2 -> MCBTripState/1
  Bus Selector/6 -> ERVRCB1-MCB/7  "<TripRequest>"
  MCBControl/1 -> Bus Selector/1
  Bus Selector/1 -> ERVRCB1-MCB/1  "<Value>"
  Bus Selector/2 -> ERVRCB1-MCB/2  "<Mode>"
  Bus Selector/3 -> ERVRCB1-MCB/3  "<InitVal>"
  Bus Selector/4 -> ERVRCB1-MCB/5  "<InternalRequest>"
  Bus Selector/5 -> ERVRCB1-MCB/6  "<Inhibit>"
  ERVRCB1-MCB/1 -> InputState/1
  Initialise/1 -> ERVRCB1-MCB/4

== system IOControls/ForEachVehicle/IOControls/Non-CabControl/CircuitBreakersofEDB/ERVRCB2 ==
  note: States:
      | Tripped
      | Set
  MCBControl : Inport  OutDataTypeStr=Bus: BD_IOControls_In_MCBControl
  Initialise : Inport  Port=2
  Bus Selector : BusSelector  OutputSignals=Value,Mode,InitVal,InternalRequest,Inhibit,TripRequest
  ERVRCB2-MCB : IOStateMachinesLib/MCB  InitSource=internal  InitState=InitState  OffStateValue=OffStateValue  OnStateValue=OnStateValue
      settings: SourceProductName=IO State Machines
  InputState : Outport  VectorParamsAs1DForOutWhenUnconnected=off
  MCBTripState : Outport  Port=2  VectorParamsAs1DForOutWhenUnconnected=off
  wires:
  ERVRCB2-MCB/2 -> MCBTripState/1
  Bus Selector/6 -> ERVRCB2-MCB/7  "<TripRequest>"
  MCBControl/1 -> Bus Selector/1
  Bus Selector/1 -> ERVRCB2-MCB/1  "<Value>"
  Bus Selector/2 -> ERVRCB2-MCB/2  "<Mode>"
  Bus Selector/3 -> ERVRCB2-MCB/3  "<InitVal>"
  Bus Selector/4 -> ERVRCB2-MCB/5  "<InternalRequest>"
  Bus Selector/5 -> ERVRCB2-MCB/6  "<Inhibit>"
  ERVRCB2-MCB/1 -> InputState/1
  Initialise/1 -> ERVRCB2-MCB/4

== system IOControls/ForEachVehicle/IOControls/Non-CabControl/CircuitBreakersofEDB/ESKCB ==
  note: States:
      | Tripped
      | Set
  MCBControl : Inport  OutDataTypeStr=Bus: BD_IOControls_In_MCBControl
  Initialise : Inport  Port=2
  Bus Selector : BusSelector  OutputSignals=Value,Mode,InitVal,InternalRequest,Inhibit,TripRequest
  ESKCB-MCB : IOStateMachinesLib/MCB  InitSource=internal  InitState=InitState  OffStateValue=OffStateValue  OnStateValue=OnStateValue
      settings: SourceProductName=IO State Machines
  InputState : Outport  VectorParamsAs1DForOutWhenUnconnected=off
  MCBTripState : Outport  Port=2  VectorParamsAs1DForOutWhenUnconnected=off
  wires:
  ESKCB-MCB/2 -> MCBTripState/1
  Bus Selector/6 -> ESKCB-MCB/7  "<TripRequest>"
  MCBControl/1 -> Bus Selector/1
  Bus Selector/1 -> ESKCB-MCB/1  "<Value>"
  Bus Selector/2 -> ESKCB-MCB/2  "<Mode>"
  Bus Selector/3 -> ESKCB-MCB/3  "<InitVal>"
  Bus Selector/4 -> ESKCB-MCB/5  "<InternalRequest>"
  Bus Selector/5 -> ESKCB-MCB/6  "<Inhibit>"
  ESKCB-MCB/1 -> InputState/1
  Initialise/1 -> ESKCB-MCB/4

== system IOControls/ForEachVehicle/IOControls/Non-CabControl/CircuitBreakersofEDB/FDSCB ==
  note: States:
      | Tripped
      | Set
  MCBControl : Inport  OutDataTypeStr=Bus: BD_IOControls_In_MCBControl
  Initialise : Inport  Port=2
  Bus Selector : BusSelector  OutputSignals=Value,Mode,InitVal,InternalRequest,Inhibit,TripRequest
  FDSCB-MCB : IOStateMachinesLib/MCB  InitSource=internal  InitState=InitState  OffStateValue=OffStateValue  OnStateValue=OnStateValue
      settings: SourceProductName=IO State Machines
  InputState : Outport  VectorParamsAs1DForOutWhenUnconnected=off
  MCBTripState : Outport  Port=2  VectorParamsAs1DForOutWhenUnconnected=off
  wires:
  FDSCB-MCB/2 -> MCBTripState/1
  Bus Selector/6 -> FDSCB-MCB/7  "<TripRequest>"
  MCBControl/1 -> Bus Selector/1
  Bus Selector/1 -> FDSCB-MCB/1  "<Value>"
  Bus Selector/2 -> FDSCB-MCB/2  "<Mode>"
  Bus Selector/3 -> FDSCB-MCB/3  "<InitVal>"
  Bus Selector/4 -> FDSCB-MCB/5  "<InternalRequest>"
  Bus Selector/5 -> FDSCB-MCB/6  "<Inhibit>"
  FDSCB-MCB/1 -> InputState/1
  Initialise/1 -> FDSCB-MCB/4

== system IOControls/ForEachVehicle/IOControls/Non-CabControl/CircuitBreakersofEDB/HCB ==
  note: States:
      | Tripped
      | Set
  MCBControl : Inport  OutDataTypeStr=Bus: BD_IOControls_In_MCBControl
  Initialise : Inport  Port=2
  Bus Selector : BusSelector  OutputSignals=Value,Mode,InitVal,InternalRequest,Inhibit,TripRequest
  HCB-MCB : IOStateMachinesLib/MCB  InitSource=internal  InitState=InitState  OffStateValue=OffStateValue  OnStateValue=OnStateValue
      settings: SourceProductName=IO State Machines
  InputState : Outport  VectorParamsAs1DForOutWhenUnconnected=off
  MCBTripState : Outport  Port=2  VectorParamsAs1DForOutWhenUnconnected=off
  wires:
  HCB-MCB/2 -> MCBTripState/1
  Bus Selector/6 -> HCB-MCB/7  "<TripRequest>"
  MCBControl/1 -> Bus Selector/1
  Bus Selector/1 -> HCB-MCB/1  "<Value>"
  Bus Selector/2 -> HCB-MCB/2  "<Mode>"
  Bus Selector/3 -> HCB-MCB/3  "<InitVal>"
  Bus Selector/4 -> HCB-MCB/5  "<InternalRequest>"
  Bus Selector/5 -> HCB-MCB/6  "<Inhibit>"
  HCB-MCB/1 -> InputState/1
  Initialise/1 -> HCB-MCB/4

== system IOControls/ForEachVehicle/IOControls/Non-CabControl/CircuitBreakersofEDB/HLLCB ==
  note: States:
      | Tripped
      | Set
  MCBControl : Inport  OutDataTypeStr=Bus: BD_IOControls_In_MCBControl
  Initialise : Inport  Port=2
  Bus Selector : BusSelector  OutputSignals=Value,Mode,InitVal,InternalRequest,Inhibit,TripRequest
  HLLCB-MCB : IOStateMachinesLib/MCB  InitSource=internal  InitState=InitState  OffStateValue=OffStateValue  OnStateValue=OnStateValue
      settings: SourceProductName=IO State Machines
  InputState : Outport  VectorParamsAs1DForOutWhenUnconnected=off
  MCBTripState : Outport  Port=2  VectorParamsAs1DForOutWhenUnconnected=off
  wires:
  HLLCB-MCB/2 -> MCBTripState/1
  Bus Selector/6 -> HLLCB-MCB/7  "<TripRequest>"
  MCBControl/1 -> Bus Selector/1
  Bus Selector/1 -> HLLCB-MCB/1  "<Value>"
  Bus Selector/2 -> HLLCB-MCB/2  "<Mode>"
  Bus Selector/3 -> HLLCB-MCB/3  "<InitVal>"
  Bus Selector/4 -> HLLCB-MCB/5  "<InternalRequest>"
  Bus Selector/5 -> HLLCB-MCB/6  "<Inhibit>"
  HLLCB-MCB/1 -> InputState/1
  Initialise/1 -> HLLCB-MCB/4

== system IOControls/ForEachVehicle/IOControls/Non-CabControl/CircuitBreakersofEDB/HLRCB ==
  note: States:
      | Tripped
      | Set
  MCBControl : Inport  OutDataTypeStr=Bus: BD_IOControls_In_MCBControl
  Initialise : Inport  Port=2
  Bus Selector : BusSelector  OutputSignals=Value,Mode,InitVal,InternalRequest,Inhibit,TripRequest
  HLRCB-MCB : IOStateMachinesLib/MCB  InitSource=internal  InitState=InitState  OffStateValue=OffStateValue  OnStateValue=OnStateValue
      settings: SourceProductName=IO State Machines
  InputState : Outport  VectorParamsAs1DForOutWhenUnconnected=off
  MCBTripState : Outport  Port=2  VectorParamsAs1DForOutWhenUnconnected=off
  wires:
  HLRCB-MCB/2 -> MCBTripState/1
  Bus Selector/6 -> HLRCB-MCB/7  "<TripRequest>"
  MCBControl/1 -> Bus Selector/1
  Bus Selector/1 -> HLRCB-MCB/1  "<Value>"
  Bus Selector/2 -> HLRCB-MCB/2  "<Mode>"
  Bus Selector/3 -> HLRCB-MCB/3  "<InitVal>"
  Bus Selector/4 -> HLRCB-MCB/5  "<InternalRequest>"
  Bus Selector/5 -> HLRCB-MCB/6  "<Inhibit>"
  HLRCB-MCB/1 -> InputState/1
  Initialise/1 -> HLRCB-MCB/4

== system IOControls/ForEachVehicle/IOControls/Non-CabControl/CircuitBreakersofEDB/HMCB ==
  note: States:
      | Tripped
      | Set
  MCBControl : Inport  OutDataTypeStr=Bus: BD_IOControls_In_MCBControl
  Initialise : Inport  Port=2
  Bus Selector : BusSelector  OutputSignals=Value,Mode,InitVal,InternalRequest,Inhibit,TripRequest
  HMCB-MCB : IOStateMachinesLib/MCB  InitSource=internal  InitState=InitState  OffStateValue=OffStateValue  OnStateValue=OnStateValue
      settings: SourceProductName=IO State Machines
  InputState : Outport  VectorParamsAs1DForOutWhenUnconnected=off
  MCBTripState : Outport  Port=2  VectorParamsAs1DForOutWhenUnconnected=off
  wires:
  HMCB-MCB/2 -> MCBTripState/1
  Bus Selector/6 -> HMCB-MCB/7  "<TripRequest>"
  MCBControl/1 -> Bus Selector/1
  Bus Selector/1 -> HMCB-MCB/1  "<Value>"
  Bus Selector/2 -> HMCB-MCB/2  "<Mode>"
  Bus Selector/3 -> HMCB-MCB/3  "<InitVal>"
  Bus Selector/4 -> HMCB-MCB/5  "<InternalRequest>"
  Bus Selector/5 -> HMCB-MCB/6  "<Inhibit>"
  HMCB-MCB/1 -> InputState/1
  Initialise/1 -> HMCB-MCB/4

== system IOControls/ForEachVehicle/IOControls/Non-CabControl/CircuitBreakersofEDB/HVAC1 ==
  note: States:
      | Tripped
      | Set
  MCBControl : Inport  OutDataTypeStr=Bus: BD_IOControls_In_MCBControl
  Initialise : Inport  Port=2
  Bus Selector : BusSelector  OutputSignals=Value,Mode,InitVal,InternalRequest,Inhibit,TripRequest
  HVAC1-MCB : IOStateMachinesLib/MCB  InitSource=internal  InitState=InitState  OffStateValue=OffStateValue  OnStateValue=OnStateValue
      settings: SourceProductName=IO State Machines
  InputState : Outport  VectorParamsAs1DForOutWhenUnconnected=off
  MCBTripState : Outport  Port=2  VectorParamsAs1DForOutWhenUnconnected=off
  wires:
  HVAC1-MCB/2 -> MCBTripState/1
  Bus Selector/6 -> HVAC1-MCB/7  "<TripRequest>"
  MCBControl/1 -> Bus Selector/1
  Bus Selector/1 -> HVAC1-MCB/1  "<Value>"
  Bus Selector/2 -> HVAC1-MCB/2  "<Mode>"
  Bus Selector/3 -> HVAC1-MCB/3  "<InitVal>"
  Bus Selector/4 -> HVAC1-MCB/5  "<InternalRequest>"
  Bus Selector/5 -> HVAC1-MCB/6  "<Inhibit>"
  HVAC1-MCB/1 -> InputState/1
  Initialise/1 -> HVAC1-MCB/4

== system IOControls/ForEachVehicle/IOControls/Non-CabControl/CircuitBreakersofEDB/HVAC2 ==
  note: States:
      | Tripped
      | Set
  MCBControl : Inport  OutDataTypeStr=Bus: BD_IOControls_In_MCBControl
  Initialise : Inport  Port=2
  Bus Selector : BusSelector  OutputSignals=Value,Mode,InitVal,InternalRequest,Inhibit,TripRequest
  HVAC2-MCB : IOStateMachinesLib/MCB  InitSource=internal  InitState=InitState  OffStateValue=OffStateValue  OnStateValue=OnStateValue
      settings: SourceProductName=IO State Machines
  InputState : Outport  VectorParamsAs1DForOutWhenUnconnected=off
  MCBTripState : Outport  Port=2  VectorParamsAs1DForOutWhenUnconnected=off
  wires:
  HVAC2-MCB/2 -> MCBTripState/1
  Bus Selector/6 -> HVAC2-MCB/7  "<TripRequest>"
  MCBControl/1 -> Bus Selector/1
  Bus Selector/1 -> HVAC2-MCB/1  "<Value>"
  Bus Selector/2 -> HVAC2-MCB/2  "<Mode>"
  Bus Selector/3 -> HVAC2-MCB/3  "<InitVal>"
  Bus Selector/4 -> HVAC2-MCB/5  "<InternalRequest>"
  Bus Selector/5 -> HVAC2-MCB/6  "<Inhibit>"
  HVAC2-MCB/1 -> InputState/1
  Initialise/1 -> HVAC2-MCB/4

== system IOControls/ForEachVehicle/IOControls/Non-CabControl/CircuitBreakersofEDB/ILCB1 ==
  note: States:
      | Tripped
      | Set
  MCBControl : Inport  OutDataTypeStr=Bus: BD_IOControls_In_MCBControl
  Initialise : Inport  Port=2
  Bus Selector : BusSelector  OutputSignals=Value,Mode,InitVal,InternalRequest,Inhibit,TripRequest
  ILCB1-MCB : IOStateMachinesLib/MCB  InitSource=internal  InitState=InitState  OffStateValue=OffStateValue  OnStateValue=OnStateValue
      settings: SourceProductName=IO State Machines
  InputState : Outport  VectorParamsAs1DForOutWhenUnconnected=off
  MCBTripState : Outport  Port=2  VectorParamsAs1DForOutWhenUnconnected=off
  wires:
  ILCB1-MCB/2 -> MCBTripState/1
  Bus Selector/6 -> ILCB1-MCB/7  "<TripRequest>"
  MCBControl/1 -> Bus Selector/1
  Bus Selector/1 -> ILCB1-MCB/1  "<Value>"
  Bus Selector/2 -> ILCB1-MCB/2  "<Mode>"
  Bus Selector/3 -> ILCB1-MCB/3  "<InitVal>"
  Bus Selector/4 -> ILCB1-MCB/5  "<InternalRequest>"
  Bus Selector/5 -> ILCB1-MCB/6  "<Inhibit>"
  ILCB1-MCB/1 -> InputState/1
  Initialise/1 -> ILCB1-MCB/4
